simulink model "PID_controller"  (R2019b)
settings: Solver=VariableStepAuto  StartTime=0.0  StopTime=60  RelTol=1e-3
values from neighbouring files (symbols this model uses):
  beta = 0.1    [PID_controller_params.m]
  Kc = 0.56    [PID_controller_params.m]    (also in PI_controller_params.m = 8)
  tau_D1 = 0.1    [PID_controller_params.m]
  tau_D2 = 1    [PID_controller_params.m]
  tau_I = 8    [PID_controller_params.m]
settings Model: Creator=adityaaaap  LastModifiedBy=adityaaaap
settings DataIOCC: ReturnWorkspaceOutputs=off
settings DebuggingCC: ArithmeticOperatorsInVariantConditions=warning
settings SFSimCC: SimUseLocalCustomCode=off  CustomCodeUndefinedFunction=UseInterfaceOnly
settings RTWCC: RTWUseLocalCustomCode=off
settings CodeAppCC: StateflowObjectComments=on

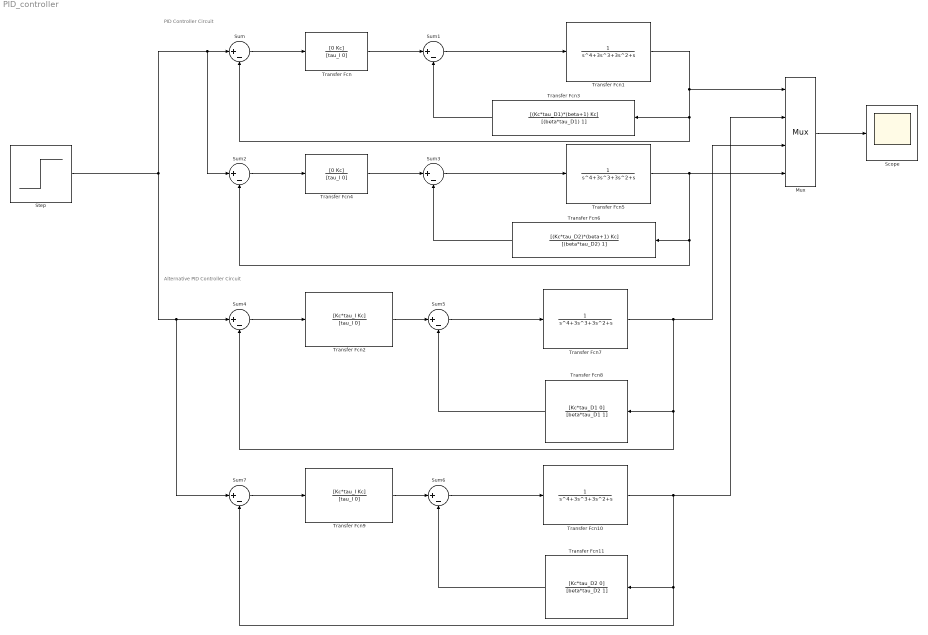
== system PID_controller ==
  note: PID Controller Circuit
  note: Alternative PID Controller Circuit
  Mux : Mux
  Scope : Scope
  Step : Step  Time=0  SampleTime=0
  Sum{,1..7} (8 alike) : Sum  Inputs=|+-
  Transfer Fcn : TransferFcn  Numerator=[0 Kc]  Denominator=[tau_I 0]
  Transfer Fcn{1,5,7,10} (4 alike) : TransferFcn  Denominator=[1 3 3 1 0]
  Transfer Fcn11 : TransferFcn  Numerator=[Kc*tau_D2 0]  Denominator=[beta*tau_D2 1]
  Transfer Fcn2 : TransferFcn  Numerator=[Kc*tau_I Kc]  Denominator=[tau_I 0]
  Transfer Fcn3 : TransferFcn  Numerator=[(Kc*tau_D1)*(beta+1) Kc]  Denominator=[(beta*tau_D1) 1]
  Transfer Fcn4 : TransferFcn  Numerator=[0 Kc]  Denominator=[tau_I 0]
  Transfer Fcn6 : TransferFcn  Numerator=[(Kc*tau_D2)*(beta+1) Kc]  Denominator=[(beta*tau_D2) 1]
  Transfer Fcn8 : TransferFcn  Numerator=[Kc*tau_D1 0]  Denominator=[beta*tau_D1 1]
  Transfer Fcn9 : TransferFcn  Numerator=[Kc*tau_I Kc]  Denominator=[tau_I 0]
  wires:
  Step/1 -> Sum7/1, Sum4/1, Sum2/1, Sum/1
  Sum/1 -> Transfer Fcn/1
  Transfer Fcn/1 -> Sum1/1
  Sum1/1 -> Transfer Fcn1/1
  Mux/1 -> Scope/1
  Transfer Fcn3/1 -> Sum1/2
  Transfer Fcn1/1 -> Sum/2, Transfer Fcn3/1, Mux/1
  Sum3/1 -> Transfer Fcn5/1
  Transfer Fcn4/1 -> Sum3/1
  Sum2/1 -> Transfer Fcn4/1
  Transfer Fcn5/1 -> Mux/4, Sum2/2, Transfer Fcn6/1
  Transfer Fcn6/1 -> Sum3/2
  Sum4/1 -> Transfer Fcn2/1
  Sum5/1 -> Transfer Fcn7/1
  Transfer Fcn2/1 -> Sum5/1
  Transfer Fcn7/1 -> Sum4/2, Transfer Fcn8/1, Mux/3
  Transfer Fcn8/1 -> Sum5/2
  Sum7/1 -> Transfer Fcn9/1
  Transfer Fcn11/1 -> Sum6/2
  Transfer Fcn9/1 -> Sum6/1
  Transfer Fcn10/1 -> Mux/2, Sum7/2, Transfer Fcn11/1
  Sum6/1 -> Transfer Fcn10/1
